simulink model "LH2Ship_Simulink_Summer"  (R2025a)
settings: Solver=VariableStepAuto  StartTime=0.0  StopTime=3600*24*7  FixedStep=0.1  MaxStep=0.5  MinStep=0.001  RelTol=1e-7  AbsTol=1e-7
values from neighbouring files (symbols this model uses):
  BoilerEff = 0.85    [PEMFC_Model.m]
  H2Consumption_kg = H2SupplyMolRate(:,1:iPmaxtot).*H2_kg_mol    [PEMFC_Model.m]
  H2Exhaust_kg = H2ExhaustMolRate(:,1:iPmaxtot).*H2_kg_mol    [PEMFC_Model.m]
  H2hhv = 141.7*10^6    (= 141700000)    [PEMFC_Model.m]
  H2lhv = 119.96*10^6    (= 119960000)    [PEMFC_Model.m]
  H2u = (0.05:0.1:0.95)    [PEMFC_Model.m]
  HeatStorageCapacity = 4.5e10    (= 45000000000)    [PEMFC_Model.m]
  HeatStorageEff = 0.9    [PEMFC_Model.m]
  HeatStorageIC = 1    [PEMFC_Model.m]
  i_FC = iCell(1,1:iPmaxtot)    [PEMFC_Model.m]
  Nstacks = 330    [PEMFC_Model.m]
  PowerElectronicsEff = 0.9    [PEMFC_Model.m]
  RecoveredHeat = NetHeatOut(:,1:iPmaxtot)    [PEMFC_Model.m]
  V_FC = Vout(:,1:iPmaxtot)    [PEMFC_Model.m]
undefined symbols (not defined in the file or in its folder): BatteryCapacity, BattInitialSOC, LH2ColdRecovery_Efficiency, LH2ColdRecovery_EnthalpyGain, mass, Rt, v, VDCBus
libraries: fl_lib x16, nesl_utility x15, simulink x5, slpidlib x2, batteryecm_lib x1, ee_lib x1
(part 2 of 2)

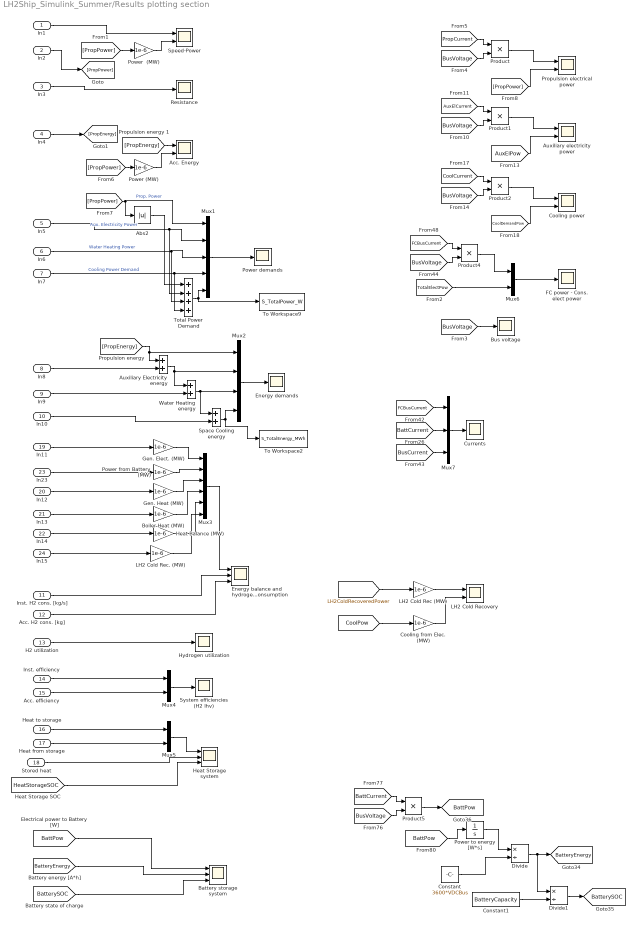
== system LH2Ship_Simulink_Summer/Results plotting section ==
  In1 : Inport
  In2 : Inport  Port=2
  In3 : Inport  Port=3
  In4 : Inport  Port=4
  In5 : Inport  Port=5
  In6 : Inport  Port=6
  In7 : Inport  Port=7
  In8 : Inport  Port=8
  In9 : Inport  Port=9
  In10 : Inport  Port=10
  Inst. H2 cons. [kg/s] : Inport  Port=11
  Acc. H2 cons. [kg] : Inport  Port=12
  H2 utilization : Inport  Port=13
  Inst. efficiency : Inport  Port=14
  Acc. efficiency : Inport  Port=15
  Heat to storage : Inport  Port=16
  Heat from storage : Inport  Port=17
  Stored heat : Inport  Port=18
  In11 : Inport  Port=19
  In12 : Inport  Port=20
  In13 : Inport  Port=21
  In14 : Inport  Port=22
  In23 : Inport  Port=23
  In15 : Inport  Port=24
  Abs2 : Abs  SaturateOnIntegerOverflow=off
  Acc. Energy : Scope  NumInputPorts=2
      settings: SampleTime=60  ActiveDisplayYMinimum=-27.73277  ActiveDisplayYMaximum=249.5949  DataLoggingVariableName=ScopeData2
  Auxiliary Electricity energy : Sum
  Auxiliary electricity power : Scope  NumInputPorts=2
      settings: SampleTime=10  ActiveDisplayYMinimum=9.70179565445E+6  ActiveDisplayYMaximum=1.286267551443E+7  DataLoggingSaveFormat=Array
  Battery storage system : Scope  NumInputPorts=3
      settings: SampleTime=20  ActiveDisplayYMinimum=-2.71505775797E+6  ActiveDisplayYMaximum=2.03600675252E+6  YLabel=Battery power flows [W] (+ charge)
  Boiler Heat (MW) : Gain  Gain=1e-6
  Bus voltage : Scope
      settings: SampleTime=15  ActiveDisplayYMinimum=95.60687  ActiveDisplayYMaximum=103.01722  DataLoggingVariableName=ScopeData2  DataLoggingSaveFormat=Array
  Constant : Constant  Value=3600*VDCBus
  Constant1 : Constant  Value=BatteryCapacity
  Cooling from Elec. (MW) : Gain  Gain=1e-6
  Cooling power : Scope  NumInputPorts=2
      settings: SampleTime=10  ActiveDisplayYMinimum=1.384819534397E+7  ActiveDisplayYMaximum=2.585953765324E+7  DataLoggingVariableName=ScopeData3  DataLoggingSaveFormat=Array
  Currents : Scope
      settings: SampleTime=10  ActiveDisplayYMinimum=-49258.9542  ActiveDisplayYMaximum=439878.56594  DataLoggingVariableName=ScopeData6  DataLoggingSaveFormat=Array
  Divide : Product  Inputs=*/
  Divide1 : Product  Inputs=*/
  Energy balance and hydrogen consumption : Scope  NumInputPorts=3
      settings: SampleTime=20  TimeUnits=Metric (based on Time Span)  ActiveDisplayString=3  ActiveDisplayYMinimum=0  ActiveDisplayYMaximum=342735.8152  YLabel=Accumulated Consumption (kg)
  Energy demands : Scope
      settings: ActiveDisplayYMinimum=-1145.91745  ActiveDisplayYMaximum=10313.25709  DataLoggingVariableName=ScopeData2
  FC power - Cons. elect power : Scope
      settings: SampleTime=20  ActiveDisplayYMinimum=2.950350565233E+7  ActiveDisplayYMaximum=3.254359686601E+7  DataLoggingVariableName=ScopeData4  DataLoggingSaveFormat=Array
  Gen. Elect. (MW) : Gain  Gain=1e-6
  Gen. Heat (MW) : Gain  Gain=1e-6
  Heat Balance (MW) : Gain  Gain=1e-6
  Heat Storage system : Scope  NumInputPorts=3
      settings: SampleTime=60  ActiveDisplayYMinimum=-5.26089937455E+6  ActiveDisplayYMaximum=1.92495802236E+6  YLabel=Heat storage flows [W]
  Hydrogen utilization : Scope
      settings: SampleTime=60  ActiveDisplayYMinimum=-0.0625  ActiveDisplayYMaximum=1.0625  YLabel=H2 Utilization
  LH2 Cold Rec (MW) : Gain  Gain=1e-6
  LH2 Cold Rec. (MW) : Gain  Gain=1e-6
  LH2 Cold Recovery : Scope  NumInputPorts=2
      settings: TimeUnits=Metric (based on Time Span)  ActiveDisplayYMinimum=0  ActiveDisplayYMaximum=12.5543  YLabel=Power (MW)  DataLoggingVariableName=ScopeData7
  Mux1 : Mux  Inputs=5
  Mux2 : Mux
  Mux3 : Mux  Inputs=6
  Mux4 : Mux  Inputs=2
  Mux5 : Mux  Inputs=2
  Mux6 : Mux  Inputs=2
  Mux7 : Mux  Inputs=3
  Power  (MW) : Gain  Gain=1e-6
  Power (MW) : Gain  Gain=1e-6
  Power demands : Scope
      settings: SampleTime=60  ActiveDisplayYMinimum=-1.024430508825E+7  ActiveDisplayYMaximum=9.219875057425E+7
  Power from Battery (MW) : Gain  Gain=1e-6
  Power to energy [W*s] : Integrator  InitialCondition=BatteryCapacity*BattInitialSOC*VDCBus*3600  LowerSaturationLimit=0
  Product{,1..2,4..5} (5 alike) : Product
  Propulsion electrical power : Scope  NumInputPorts=2
      settings: SampleTime=10  ActiveDisplayYMinimum=1.953373799458E+7  ActiveDisplayYMaximum=2.207089058064E+7  DataLoggingVariableName=ScopeData5  DataLoggingSaveFormat=Array
  Resistance : Scope
      settings: SampleTime=60  ActiveDisplayYMinimum=-292626.05775  ActiveDisplayYMaximum=2.63328258101E+6
  Space Cooling energy : Sum
  Speed-Power : Scope  NumInputPorts=2
      settings: SampleTime=60  ActiveDisplayYMinimum=-2.66774  ActiveDisplayYMaximum=20.24561
  System efficiencies (H2 lhv) : Scope
      settings: SampleTime=60  ActiveDisplayYMinimum=-0.17169  ActiveDisplayYMaximum=1.54521  YLabel=System efficiency
  To Workspace2 : ToWorkspace  VariableName=S_TotalEnergy_MWh  SampleTime=30
  To Workspace9 : ToWorkspace  VariableName=S_TotalPower_W  SampleTime=30
  Total Power Demand : Sum  Inputs=++++
  Water Heating energy : Sum
  tag scope: BattPow=global, BatteryEnergy=global, BatterySOC=global
  wires:
  Mux4/1 -> System efficiencies (H2 lhv)/1
  In5/1 -> Mux1/2, Total Power Demand/2  "Aux. Electricity Power"
  Auxiliary Electricity energy/1 -> Water Heating energy/1, Mux2/2
  In9/1 -> Water Heating energy/2
  Acc. efficiency/1 -> Mux4/2
  In6/1 -> Mux1/3, Total Power Demand/3  "Water Heating Power"
  Total Power Demand/1 -> To Workspace9/1, Mux1/5
  Power  (MW)/1 -> Speed-Power/2
  Mux5/1 -> Heat Storage system/1
  [PropPower] -> Mux1/1, Abs2/1  "Prop. Power"
  Abs2/1 -> Total Power Demand/1
  [PropPower] -> Power (MW)/1
  [PropEnergy] -> Auxiliary Electricity energy/1, Mux2/1
  Mux2/1 -> Energy demands/1
  Water Heating energy/1 -> Mux2/3, Space Cooling energy/1
  Space Cooling energy/1 -> To Workspace2/1, Mux2/4
  In7/1 -> Total Power Demand/4, Mux1/4  "Cooling Power Demand"
  Mux1/1 -> Power demands/1
  Power (MW)/1 -> Acc. Energy/2
  Stored heat/1 -> Heat Storage system/2
  Inst. efficiency/1 -> Mux4/1
  Acc. H2 cons. [kg]/1 -> Energy balance and hydrogen consumption/3
  Heat to storage/1 -> Mux5/1
  Heat from storage/1 -> Mux5/2
  In8/1 -> Auxiliary Electricity energy/2
  In3/1 -> Resistance/1
  Inst. H2 cons. [kg/s]/1 -> Energy balance and hydrogen consumption/2
  H2 utilization/1 -> Hydrogen utilization/1
  In10/1 -> Space Cooling energy/2
  In1/1 -> Speed-Power/1
  In2/1 -> [PropPower]
  [PropPower] -> Power  (MW)/1
  In4/1 -> [PropEnergy]
  [PropEnergy] -> Acc. Energy/1
  In23/1 -> Power from Battery (MW)/1
  Gen. Heat (MW)/1 -> Mux3/3
  Mux3/1 -> Energy balance and hydrogen consumption/1
  Boiler Heat (MW)/1 -> Mux3/4
  In14/1 -> Heat Balance (MW)/1
  Power from Battery (MW)/1 -> Mux3/2
  In11/1 -> Gen. Elect. (MW)/1
  In13/1 -> Boiler Heat (MW)/1
  Gen. Elect. (MW)/1 -> Mux3/1
  Heat Balance (MW)/1 -> Mux3/5
  In12/1 -> Gen. Heat (MW)/1
  [BattPow] -> Battery storage system/1
  [BatteryEnergy] -> Battery storage system/2
  [BatterySOC] -> Battery storage system/3
  [HeatStorageSOC] -> Heat Storage system/3
  [TotalElectPow] -> Mux6/2
  Mux6/1 -> FC power - Cons. elect power/1
  Product1/1 -> Auxiliary electricity power/1
  [PropCurrent] -> Product/1
  [BusVoltage] -> Product1/2
  [CoolDemandPow] -> Cooling power/2
  [BusVoltage] -> Product/2
  [PropPower] -> Propulsion electrical power/2
  [BusVoltage] -> Bus voltage/1
  Product2/1 -> Cooling power/1
  [CoolCurrent] -> Product2/1
  [AuxElPow] -> Auxiliary electricity power/2
  [FCBusCurrent] -> Product4/1
  [AuxElCurrent] -> Product1/1
  [BusVoltage] -> Product2/2
  [BusVoltage] -> Product4/2
  Product/1 -> Propulsion electrical power/1
  Product4/1 -> Mux6/1
  Divide1/1 -> [BatterySOC]
  Divide/1 -> Divide1/1, [BatteryEnergy]
  Power to energy [W*s]/1 -> Divide/1
  Mux7/1 -> Currents/1
  [FCBusCurrent] -> Mux7/1
  [BattCurrent] -> Product5/1
  Constant1/1 -> Divide1/2
  Product5/1 -> [BattPow]
  [BattCurrent] -> Mux7/2
  [BusCurrent] -> Mux7/3
  Constant/1 -> Divide/2
  [BattPow] -> Power to energy [W*s]/1
  [BusVoltage] -> Product5/2
  In15/1 -> LH2 Cold Rec. (MW)/1
  LH2 Cold Rec. (MW)/1 -> Mux3/6
  [LH2ColdRecoveredPower] -> LH2 Cold Rec (MW)/1
  [CoolPow] -> Cooling from Elec. (MW)/1
  LH2 Cold Rec (MW)/1 -> LH2 Cold Recovery/1
  Cooling from Elec. (MW)/1 -> LH2 Cold Recovery/2

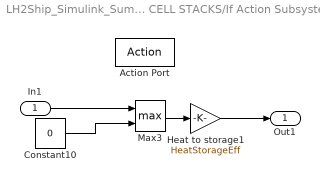
== system LH2Ship_Simulink_Summer/PEM FUEL CELL STACKS/If Action Subsystem ==
  In1 : Inport
  Action Port : ActionPort  ActionPortLabel=if(u1 > 0)
  Constant10 : Constant  Value=0
  Heat to storage1 : Gain  Gain=HeatStorageEff
  Max3 : MinMax  Function=max  Inputs=2
  Out1 : Outport  VectorParamsAs1DForOutWhenUnconnected=off
  wires:
  Constant10/1 -> Max3/2
  In1/1 -> Max3/1
  Max3/1 -> Heat to storage1/1
  Heat to storage1/1 -> Out1/1

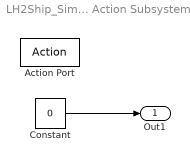
== system LH2Ship_Simulink_Summer/PEM FUEL CELL STACKS/If Action Subsystem1 ==
  Action Port : ActionPort  ActionPortLabel=else
  Constant : Constant  Value=0
  Out1 : Outport  VectorParamsAs1DForOutWhenUnconnected=off
  wires:
  Constant/1 -> Out1/1

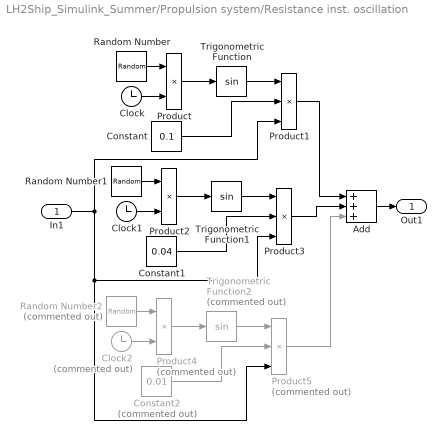
== system LH2Ship_Simulink_Summer/Propulsion system/Resistance inst. oscillation ==
  In1 : Inport
  Add : Sum  Inputs=3
  Clock : Clock
  Clock1 : Clock
  Clock2 : Clock  Commented=on
  Constant : Constant  Value=0.1
  Constant1 : Constant  Value=0.04
  Constant2 : Constant  Commented=on  Value=0.01
  Product : Product
  Product1 : Product  Inputs=3
  Product2 : Product
  Product3 : Product  Inputs=3
  Product4 : Product  Commented=on
  Product5 : Product  Commented=on  Inputs=3
  Random Number : RandomNumber  Mean=pi/1000000  Variance=0.00000005  Seed=0.00005  SampleTime=100
  Random Number1 : RandomNumber  Mean=pi/6  Variance=0.5  Seed=0.3  SampleTime=200
  Random Number2 : RandomNumber  Commented=on  Mean=pi  Variance=3  Seed=3  SampleTime=10
  Trigonometric Function : Trigonometry
  Trigonometric Function1 : Trigonometry
  Trigonometric Function2 : Trigonometry  Commented=on
  Out1 : Outport  VectorParamsAs1DForOutWhenUnconnected=off
  wires:
  Clock2/1 -> Product4/2
  Clock/1 -> Product/2
  Product4/1 -> Trigonometric Function2/1
  Constant/1 -> Product1/2
  Clock1/1 -> Product2/2
  Product/1 -> Trigonometric Function/1
  In1/1 -> Product5/3, Product3/3, Product1/3
  Product5/1 -> Add/3
  Product1/1 -> Add/1
  Trigonometric Function1/1 -> Product3/1
  Constant1/1 -> Product3/2
  Product2/1 -> Trigonometric Function1/1
  Random Number1/1 -> Product2/1
  Constant2/1 -> Product5/2
  Trigonometric Function/1 -> Product1/1
  Random Number/1 -> Product/1
  Add/1 -> Out1/1
  Product3/1 -> Add/2
  Trigonometric Function2/1 -> Product5/1
  Random Number2/1 -> Product4/1
